simulink model "simModel_open_loop_systems"  (R2025b)
settings: Solver=FixedStepAuto  StartTime=0.0  StopTime=10.0  FixedStep=0.001  RelTol=1e-3
InitFcn:
  | load data\FC1.mat
  | load data\FC2.mat
  | load data\FC3.mat
  | load data\FC4.mat
undefined symbols (not defined in the file or in its folder): FC1, FC2, FC3, FC4
libraries: simulink_extras x4
settings Model: Creator=ismet  LastModifiedBy=ismet

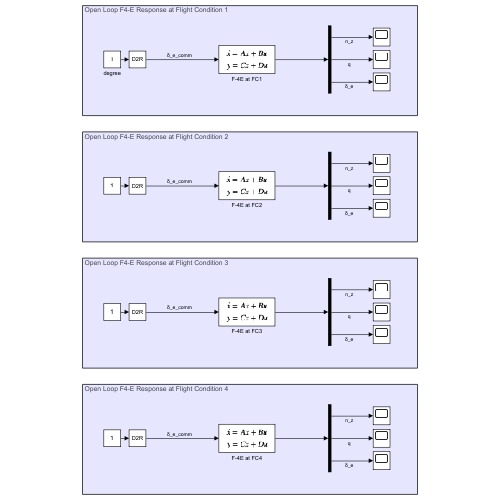
[thumbnail: Simulink's stored preview of the top-level diagram]
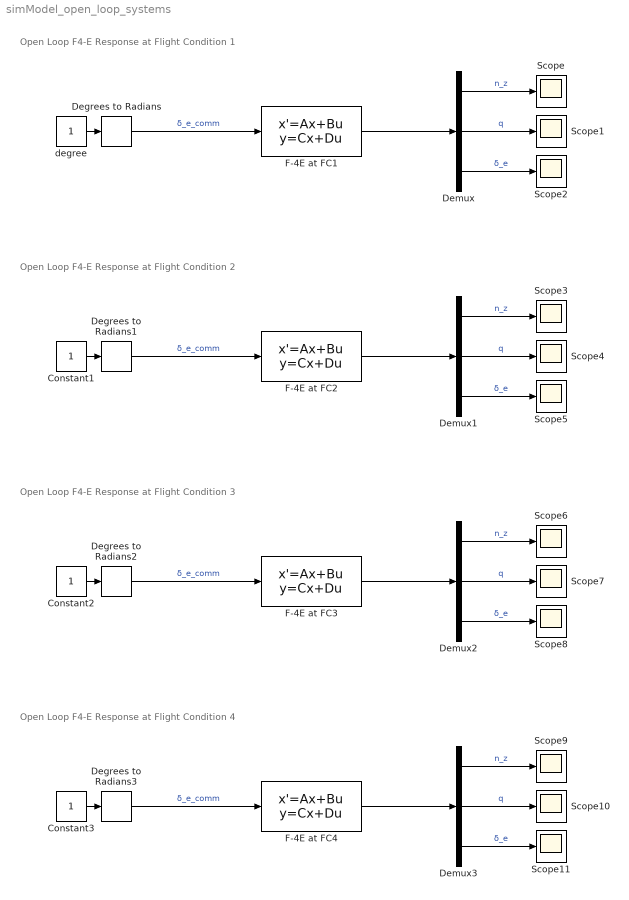
== system simModel_open_loop_systems ==
  note: Open Loop F4-E Response at Flight Condition 1
  note: Open Loop F4-E Response at Flight Condition 2
  note: Open Loop F4-E Response at Flight Condition 3
  note: Open Loop F4-E Response at Flight Condition 4
  Constant1 : Constant
  Constant2 : Constant
  Constant3 : Constant
  Degrees to Radians{,1..3} (4 alike) : simulink_extras/Transformations/Degrees to Radians
  Demux{,1..3} (4 alike) : Demux  Outputs=3
  F-4E at FC1 : StateSpace  A=FC1.A  B=FC1.B  C=FC1.C  D=FC1.D  InitialCondition=0  ContinuousStateAttributes=['n_z', 'q', 'delta_e']
  F-4E at FC2 : StateSpace  A=FC2.A  B=FC2.B  C=FC2.C  D=FC2.D  InitialCondition=0  ContinuousStateAttributes=['n_z', 'q', 'delta_e']
  F-4E at FC3 : StateSpace  A=FC3.A  B=FC3.B  C=FC3.C  D=FC3.D  InitialCondition=0  ContinuousStateAttributes=['n_z', 'q', 'delta_e']
  F-4E at FC4 : StateSpace  A=FC4.A  B=FC4.B  C=FC4.C  D=FC4.D  InitialCondition=0  ContinuousStateAttributes=['n_z', 'q', 'delta_e']
  Scope{,1..11} (12 alike) : Scope
      Scope settings: ActiveDisplayYMinimum=-161507.34984355632  ActiveDisplayYMaximum=17945.261093728477
      Scope10 settings: ActiveDisplayYMinimum=-0.086341754821145075  ActiveDisplayYMaximum=0.026016643527915575  DataLoggingVariableName=ScopeData9
      Scope11 settings: DataLoggingVariableName=ScopeData10
      Scope2 settings: ActiveDisplayYMinimum=-0.0021816615649928963  ActiveDisplayYMaximum=0.019634954084936072  DataLoggingVariableName=ScopeData2
      Scope3 settings: ActiveDisplayYMinimum=-1.4411398585763451E+8  ActiveDisplayYMaximum=1.6012665095292721E+7  DataLoggingVariableName=ScopeData3
      Scope4 settings: DataLoggingVariableName=ScopeData4
      Scope5 settings: DataLoggingVariableName=ScopeData5
      Scope6 settings: ActiveDisplayYMinimum=-722.37831659731773  ActiveDisplayYMaximum=80.264257399701961  DataLoggingVariableName=ScopeData6
      Scope7 settings: DataLoggingVariableName=ScopeData7
      Scope8 settings: DataLoggingVariableName=ScopeData8
      Scope9 settings: ActiveDisplayYMinimum=-1.1280386882368523  ActiveDisplayYMaximum=0.1253376320263169  DataLoggingVariableName=ScopeData11
  degree : Constant
  wires:
  degree/1 -> Degrees to Radians/1
  Degrees to Radians/1 -> F-4E at FC1/1  "δ_e_comm"
  F-4E at FC1/1 -> Demux/1
  Demux/1 -> Scope/1  "n_z"
  Demux/2 -> Scope1/1  "q"
  Demux/3 -> Scope2/1  "δ_e"
  F-4E at FC2/1 -> Demux1/1
  Constant1/1 -> Degrees to Radians1/1
  Demux1/1 -> Scope3/1  "n_z"
  Demux1/3 -> Scope5/1  "δ_e"
  Demux1/2 -> Scope4/1  "q"
  Degrees to Radians1/1 -> F-4E at FC2/1  "δ_e_comm"
  Demux2/1 -> Scope6/1  "n_z"
  Constant2/1 -> Degrees to Radians2/1
  Demux2/3 -> Scope8/1  "δ_e"
  Demux2/2 -> Scope7/1  "q"
  F-4E at FC3/1 -> Demux2/1
  Degrees to Radians2/1 -> F-4E at FC3/1  "δ_e_comm"
  Demux3/1 -> Scope9/1  "n_z"
  Degrees to Radians3/1 -> F-4E at FC4/1  "δ_e_comm"
  Demux3/2 -> Scope10/1  "q"
  F-4E at FC4/1 -> Demux3/1
  Demux3/3 -> Scope11/1  "δ_e"
  Constant3/1 -> Degrees to Radians3/1
